simulink model "festotemplate"  (R2021b)
settings: Solver=ode45  StartTime=0.0  StopTime=10  RelTol=1e-3  EnableMultiTasking=on
InitFcn:
  | hwinit
values from neighbouring files (symbols this model uses):
  adingain = [1 lasergain  encodergain 1 1 1 1]    [hwinit.m]
  adinoffs = [0 laseroffset encoderoffset 0 0 0 0]    [hwinit.m]
  adoutoff = -0.19    [hwinit.m]
  Akg = Anew-L*Cnew    [NewModel.m]    (also in RunFinalExperiments.m = Anew - L*Cnew; RunFinalExperimentsLQG.m = Anew - L*Cnew; RunFromMatlab.m)
  Bkg = [Bnew L]    [NewModel.m]    (also in RunFinalExperiments.m = [Bnew, L]; RunFinalExperimentsLQG.m = [Bnew, L]; RunFromMatlab.m)
  Ckg = eye(3)    [NewModel.m]    (also in RunFinalExperiments.m; RunFinalExperimentsLQG.m; RunFromMatlab.m)
  Dkg = 0*[Bnew L]    [NewModel.m]    (also in RunFinalExperiments.m = zeros(3, 4); RunFinalExperimentsLQG.m = zeros(3, 4); RunFromMatlab.m)
  h = 1e-3    (= 0.001)    [DampingExperiments.m]    (also in FindDamping.m; FindResonance.m; HinfRunFromMatlab.m; Hinfmodel.m)
  Klqr = [-4.7204e+02, -2.4792e+01, 2.4350e+01]    [RunFinalExperiments.m]    (also in RunFinalExperimentsLQG.m = [0 0 0]; RunFromMatlab.m = [-4.7204e+02  -2.4792e+01   2.4350e+01])
libraries: eeGeneralControl x2, simulink x1
settings Model: Creator=rbabuska  LastModifiedBy=wsboer
settings SolverCC: AlgebraicLoopSolver=TrustRegion
settings DataIOCC: LimitDataPoints=on  SaveFormat=Array  ReturnWorkspaceOutputs=off  SignalLoggingName=sigsOut
settings OptimizationCC: BooleanDataType=off  ExpressionDepthLimit=2147483647  InitFltsAndDblsToZero=on  LifeSpan=inf
settings DebuggingCC: SaveWithParameterizedLinksMsg=none  SignalResolutionControl=TryResolveAllWithWarning  MultiTaskDSMMsg=warning  MultiTaskCondExecSysMsg=none  AllowSymbolicDim=off  StateNameClashWarn=warning  SFUnexpectedBacktrackingDiag=warning  SFNoUnconditionalDefaultTransitionDiag=warning  SFExecutionAtInitializationDiag=none  SFMachineParentedDataDiag=warning  ArithmeticOperatorsInVariantConditions=warning
settings HardwareCC: ProdBitPerPointer=32  ProdBitPerSizeT=32  ProdBitPerPtrDiffT=32  ProdLargestAtomicFloat=None  ProdIntDivRoundTo=Undefined  ProdEndianess=Unspecified  ProdWordSize=32  ProdHWDeviceType=32-bit Generic  TargetUnknown=on
settings ModelReferenceCC: PropagateSignalLabelsOutOfModel=off
settings SFSimCC: SimUseLocalCustomCode=off  CustomCodeUndefinedFunction=UseInterfaceOnly
settings RTWCC: RTWUseLocalCustomCode=off
settings CodeAppCC: StateflowObjectComments=on
settings GRTTargetCC: TargetFcnLib=ansi_tfl_tmw.mat  TargetLangStandard=C89/C90 (ANSI)  CombineOutputUpdateFcns=off  GRTInterface=on
settings ConfigComp: CovMetricSettings=dw  CovSaveCumulativeToWorkspaceVar=on  CovSaveSingleToWorkspaceVar=on  CovExternalEMLEnable=off

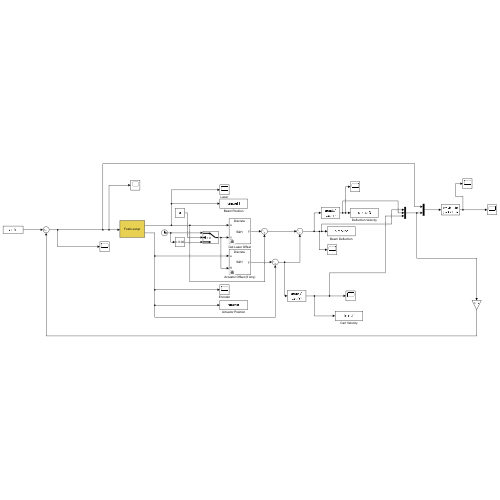
[thumbnail: Simulink's stored preview of the top-level diagram]
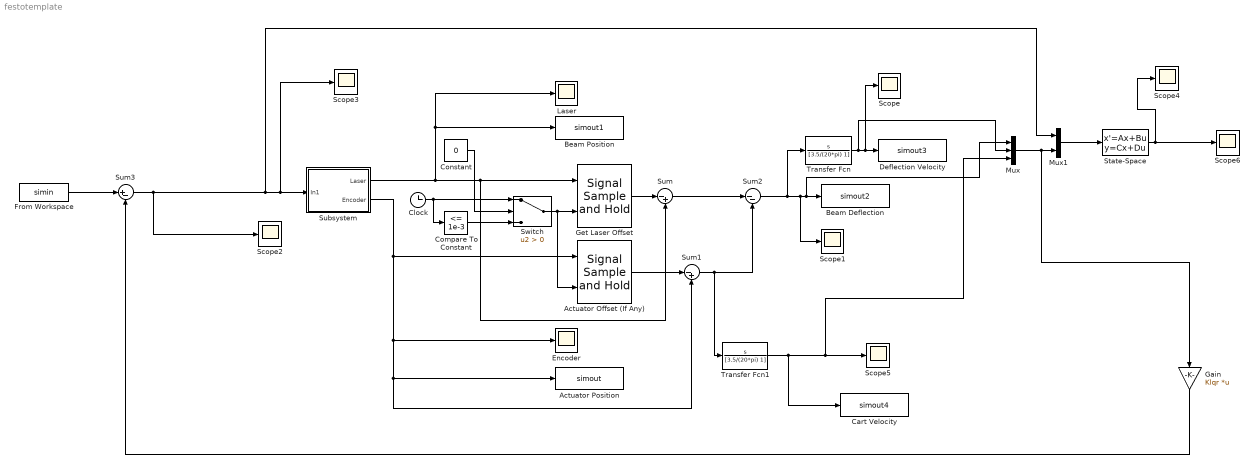
== system festotemplate ==
  Actuator Offset (If Any) : eeGeneralControl/Signal Sample and Hold  LabelModeActiveChoice=Discrete  x0=0  Ts=-1
      settings: SourceProductBaseCode=PS
  Actuator Position : ToWorkspace  VariableName=simout  SaveFormat=Timeseries  SampleTime=h
  Beam Deflection : ToWorkspace  VariableName=simout2  SaveFormat=Timeseries  SampleTime=-1
  Beam Position : ToWorkspace  VariableName=simout1  SaveFormat=Timeseries  SampleTime=h
  Cart Velocity : ToWorkspace  VariableName=simout4  SaveFormat=Timeseries  SampleTime=-1
  Clock : Clock
  Compare To Constant : simulink/Logic and Bit Operations/Compare To Constant  relop=<=  const=1e-3  OutDataTypeStr=uint8
  Constant : Constant  Value=0
  Deflection Velocity : ToWorkspace  VariableName=simout3  SaveFormat=Timeseries  SampleTime=-1
  Encoder : Scope
  From Workspace : FromWorkspace  VariableName=simin
  Gain : Gain  Gain=Klqr  Multiplication=Matrix(K*u)
  Get Laser Offset : eeGeneralControl/Signal Sample and Hold  LabelModeActiveChoice=Discrete  x0=0  Ts=-1
      settings: SourceProductBaseCode=PS
  Laser : Scope
  Mux : Mux  Inputs=3
  Mux1 : Mux  Inputs=2
  Scope{,1..6} (7 alike) : Scope
  State-Space : StateSpace  A=Akg  B=Bkg  C=Ckg  D=Dkg  InitialCondition=0
  Subsystem : Subsystem
      mask Display: disp('Festo setup')
  Sum : Sum  Inputs=|-+
  Sum1 : Sum  Inputs=|-+
  Sum2 : Sum  Inputs=|--
  Sum3 : Sum  Inputs=|+-
  Switch : Switch  Criteria=u2 > Threshold
  Transfer Fcn : TransferFcn  Numerator=[1 0]  Denominator=[3.5/(20*pi) 1]
  Transfer Fcn1 : TransferFcn  Numerator=[1 0]  Denominator=[3.5/(20*pi) 1]
  wires:
  Subsystem/2(Encoder) -> Actuator Offset (If Any)/1, Sum1/2, Actuator Position/1, Encoder/1
  Subsystem/1(Laser) -> Laser/1, Beam Position/1, Sum/2, Get Laser Offset/1
  Clock/1 -> Switch/1, Compare To Constant/1
  Compare To Constant/1 -> Switch/3
  Switch/1 -> Actuator Offset (If Any)/2, Get Laser Offset/2
  Get Laser Offset/1 -> Sum/1
  Actuator Offset (If Any)/1 -> Sum1/1
  Sum/1 -> Sum2/1
  Sum1/1 -> Transfer Fcn1/1, Sum2/2
  Sum2/1 -> Transfer Fcn/1, Scope1/1, Mux/1, Beam Deflection/1
  From Workspace/1 -> Sum3/1
  Mux1/1 -> State-Space/1
  Mux/1 -> Gain/1, Mux1/2
  State-Space/1 -> Scope6/1, Scope4/1
  Gain/1 -> Sum3/2
  Sum3/1 -> Mux1/1, Scope3/1, Subsystem/1(In1), Scope2/1
  Constant/1 -> Switch/2
  Transfer Fcn1/1 -> Cart Velocity/1, Mux/3, Scope5/1
  Transfer Fcn/1 -> Mux/2, Deflection Velocity/1, Scope/1

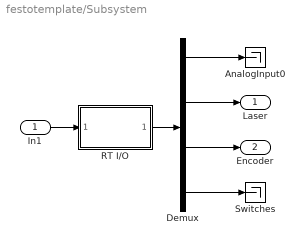
== system festotemplate/Subsystem ==
  In1 : Inport
  AnalogInput0 : Terminator
  Demux : Demux  Outputs=[1 1 1 4]
  RT I/O : Subsystem  mask{Ts=h, channels=[6 7 3]}
      mask prompts: Ts "Sample time [s]:"; channels "The 3 channels to read (e.g. [6 7 3])"
      mask init:
      | hwinit;
      | 
      | % initialize FPGA
      | fugihandle = fugiboard('Open', 'Pendulum1');
      | fugihandle.WatchdogTimeout = 0.5;
      | fugiboard('SetParams', fugihandle);
      | fugiboard('Write', fugihandle, 0, 0, 0, 0);  % dummy write to sync interface board
      | fugiboard('Write', fugihandle, 5, 1, 0, 0);  % reset position, activate relay
      | data = fugiboard('Read', fugihandle);        % get version info from FPGA
      | % model = bitshift(data(1), -5); 
      | % version = bitand(data(1), 31);
      | % disp(sprintf('FPGA setup %d, version %d', model, version)); % for the B&P it should say 1 1, or else there is a problem
      | fugiboard('Write', fugihandle, 0, 1, 0, 0);  % end reset
      | pause(0.1);                         % give relay some time to respond
      mask Display: disp('Flexible\nBeam')
  Switches : Terminator
  Laser : Outport
  Encoder : Outport  Port=2
  wires:
  RT I/O/1(Outputs) -> Demux/1
  In1/1 -> RT I/O/1(Motors)
  Demux/2 -> Laser/1
  Demux/1 -> AnalogInput0/1
  Demux/3 -> Encoder/1
  Demux/4 -> Switches/1

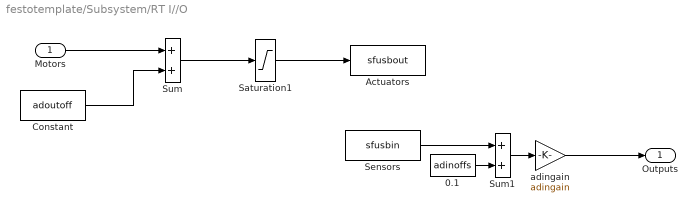
== system festotemplate/Subsystem/RT I//O ==
  Motors : Inport
  0.1 : Constant  Value=adinoffs
  Actuators : S-Function  FunctionName=sfusbout  Parameters=Ts, fugihandle  SFunctionDeploymentMode=off  EnableBusSupport=off
  Constant : Constant  Value=adoutoff
  Saturation1 : Saturate  UpperLimit=10  LowerLimit=-10
  Sensors : S-Function  FunctionName=sfusbin  Parameters=Ts, fugihandle, channels  SFunctionDeploymentMode=off  EnableBusSupport=off
  Sum : Sum  InputSameDT=on  SaturateOnIntegerOverflow=on  OutDataTypeStr=Inherit: Same as first input
  Sum1 : Sum  InputSameDT=on  SaturateOnIntegerOverflow=on  OutDataTypeStr=Inherit: Same as first input
  adingain : Gain  Gain=adingain  SaturateOnIntegerOverflow=on  OutDataTypeStr=Inherit: Same as input  ParamDataTypeStr=Inherit: Same as input
  Outputs : Outport
  wires:
  Motors/1 -> Sum/1
  Sum1/1 -> adingain/1
  0.1/1 -> Sum1/2
  Sensors/1 -> Sum1/1
  adingain/1 -> Outputs/1
  Saturation1/1 -> Actuators/1
  Sum/1 -> Saturation1/1
  Constant/1 -> Sum/2
